simulink model "pvpanelPaper_1"  (R2020a)
settings: Solver=ode45  StartTime=0.0  StopTime=10.0  RelTol=1e-3  EnableMultiTasking=on
settings Model: Creator=shrad  LastModifiedBy=shrad
settings DataIOCC: LimitDataPoints=on  SaveFormat=Array  ReturnWorkspaceOutputs=off
settings OptimizationCC: LifeSpan=inf
settings DebuggingCC: SFUnexpectedBacktrackingDiag=warning  SFNoUnconditionalDefaultTransitionDiag=warning  SFExecutionAtInitializationDiag=none  ArithmeticOperatorsInVariantConditions=warning
settings HardwareCC: ProdBitPerPointer=32  ProdBitPerSizeT=32  ProdBitPerPtrDiffT=32  ProdLargestAtomicFloat=None  ProdIntDivRoundTo=Undefined  ProdEndianess=Unspecified  ProdWordSize=32  ProdHWDeviceType=32-bit Generic
settings ModelReferenceCC: PropagateSignalLabelsOutOfModel=off
settings SFSimCC: SimUseLocalCustomCode=off  CustomCodeUndefinedFunction=UseInterfaceOnly
settings RTWCC: RTWUseLocalCustomCode=off
settings CodeAppCC: StateflowObjectComments=on
settings GRTTargetCC: TargetLangStandard=C89/C90 (ANSI)
settings ConfigComp: CovMetricSettings=dw  CovHtmlReporting=on  CovSaveCumulativeToWorkspaceVar=on  CovSaveSingleToWorkspaceVar=on  CovExternalEMLEnable=off

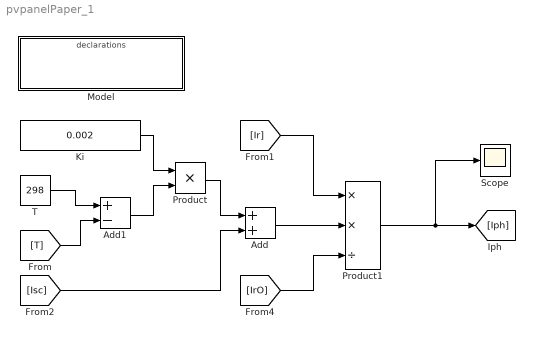
== system pvpanelPaper_1 ==
  Add : Sum
  Add1 : Sum  Inputs=+-
  Ki : Constant  Value=0.002
  Model : ModelReference  ModelNameDialog=declarations.slx  SimulationMode=Normal  ModelReferenceVersion=1.1
  Product : Product
  Product1 : Product  Inputs=**/
  Scope : Scope
  T : Constant  Value=298
  wires:
  Ki/1 -> Product/1
  Product/1 -> Add/1
  [Isc] -> Add/2
  Add/1 -> Product1/2
  [Ir] -> Product1/1
  Product1/1 -> Scope/1, [Iph]
  [T] -> Add1/2
  T/1 -> Add1/1
  Add1/1 -> Product/2
  [IrO] -> Product1/3
